simulink model "MOdel"  (R2019a)
settings: Solver=VariableStepAuto  StartTime=0.0  StopTime=30  RelTol=1e-3
libraries: simulink x2, vrlib x2, mpcadaslib x1
settings Model: Creator=pawar  LastModifiedBy=pawar

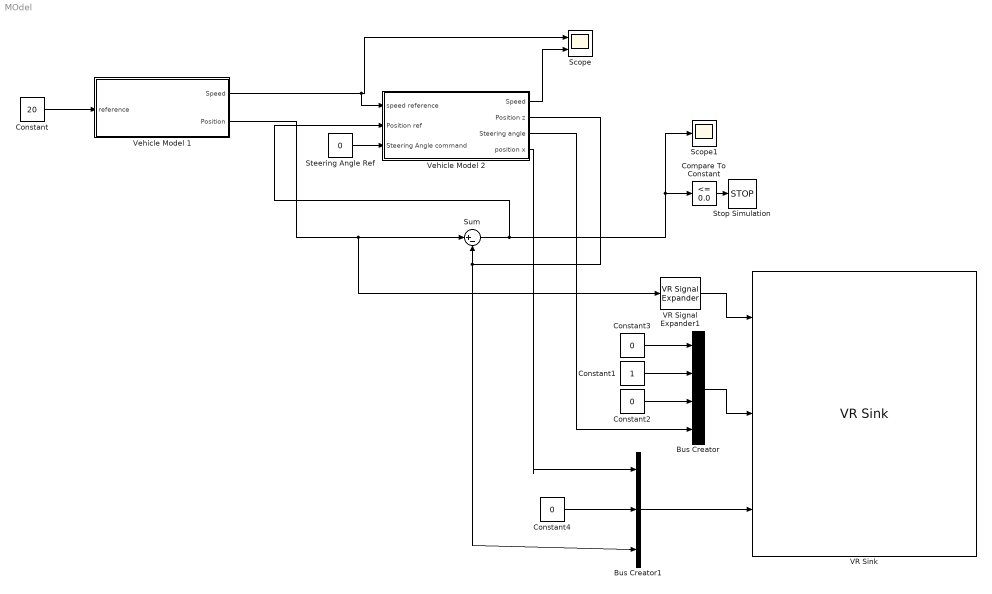
== system MOdel ==
  Bus Creator : BusCreator  Inputs=4
  Bus Creator1 : BusCreator  Inputs=3
  Compare To Constant : simulink/Logic and Bit Operations/Compare To Constant  relop=<=  const=0.0  OutDataTypeStr=boolean
  Constant : Constant  Value=20
  Constant1 : Constant
  Constant2 : Constant  Value=0
  Constant3 : Constant  Value=0
  Constant4 : Constant  Value=0
  Scope : Scope  NumInputPorts=2
  Scope1 : Scope
  Steering Angle Ref : Constant  Value=0
  Stop Simulation : Stop
  Sum : Sum  Inputs=|+-
  VR Signal Expander1 : vrlib/VR Signal Expander  outwidth=3  outidx=[3]
      settings: SourceProductName=Simulink
  VR Sink : vrlib/VR Sink  InstantiateOnLoad=on  SampleTime=0.1  ViewEnable=on  RemoteChange=off  RemoteView=off  FieldsWritten=Car_Red.translation.3.1.1.double#Car_Blue.rotation.4.1.1.double#Car_Blue.translation.3.1.1.double  WorldFileName=PlatoonWorld.WRL  AutoView=off  VideoDimensions=[]  AllowVariableSize=off
      settings: SourceProductName=Simulink
  Vehicle Model 1 : Subsystem  mask{Parameter3=[], Value=10, Value_1=20}
      mask prompts: Value "Initial Speed"; Value_1 "Initail Position"
      mask TypeOptions Value:
      | Initial Speed
      | /Value
      mask TypeOptions Value_1: Initial Position/Value
  Vehicle Model 2 : Subsystem  mask{Parameter3=[], Value=5, V=0}
      mask prompts: Value "Initial Speed"; V "Initial Position"
      mask TypeOptions Value:
      | Initial Speed
      | /Value
      mask TypeOptions V: Initial Position z/Value
  wires:
  Constant/1 -> Vehicle Model 1/1(reference)
  Vehicle Model 1/1(Speed) -> Vehicle Model 2/1(speed reference), Scope/1
  Vehicle Model 1/2("Position ") -> VR Signal Expander1/1, Sum/1
  Vehicle Model 2/1(Speed) -> Scope/2
  Vehicle Model 2/2("Position z ") -> Bus Creator1/3, Sum/2
  Sum/1 -> Vehicle Model 2/2("Position ref "), Compare To Constant/1, Scope1/1
  Compare To Constant/1 -> Stop Simulation/1
  Steering Angle Ref/1 -> Vehicle Model 2/3(Steering Angle command)
  VR Signal Expander1/1 -> VR Sink/1
  Bus Creator1/1 -> VR Sink/3
  Vehicle Model 2/3(Steering angle) -> Bus Creator/4
  Bus Creator/1 -> VR Sink/2
  Constant1/1 -> Bus Creator/2
  Constant3/1 -> Bus Creator/1
  Constant2/1 -> Bus Creator/3
  Constant4/1 -> Bus Creator1/2
  Vehicle Model 2/4(position x) -> Bus Creator1/1

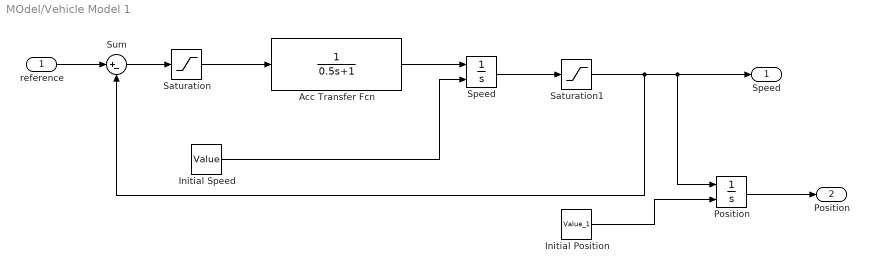
== system MOdel/Vehicle Model 1 ==
  reference : Inport
  Acc Transfer Fcn : TransferFcn  Denominator=[0.5 1]
  Initial Position : Constant  Value=Value_1
  "Initial Speed " : Constant  Value=Value
  Position : Integrator  InitialConditionSource=external
  Saturation : Saturate  UpperLimit=2  LowerLimit=-3
  Saturation1 : Saturate  UpperLimit=inf  LowerLimit=0
  "Speed " : Integrator  InitialConditionSource=external
  Sum : Sum  Inputs=|+-
  Speed : Outport
  "Position " : Outport  Port=2
  wires:
  Saturation1/1 -> Sum/2, Speed/1, Position/1
  Saturation/1 -> Acc Transfer Fcn/1
  "Initial Speed "/1 -> "Speed "/2
  Position/1 -> "Position "/1
  Sum/1 -> Saturation/1
  reference/1 -> Sum/1
  Acc Transfer Fcn/1 -> "Speed "/1
  Initial Position/1 -> Position/2
  "Speed "/1 -> Saturation1/1

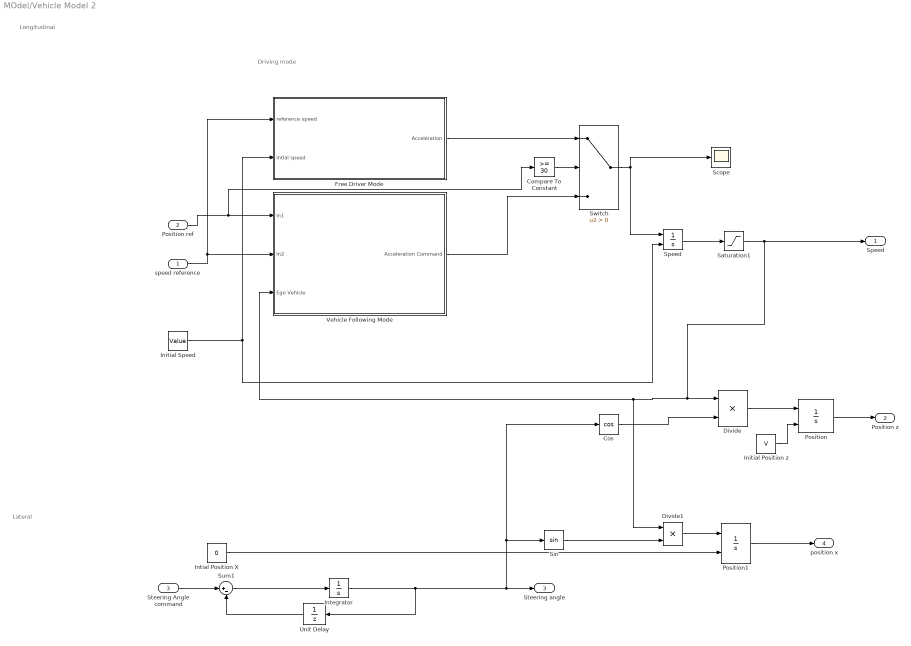
== system MOdel/Vehicle Model 2 ==
  note: Driving mode
  note: Lateral
  note: Longitudinal
  speed reference : Inport
  "Position ref " : Inport  Port=2
  Steering Angle command : Inport  Port=3
  Compare To Constant : simulink/Logic and Bit Operations/Compare To Constant  relop=>=  const=30  OutDataTypeStr=boolean
  Cos : Trigonometry  Operator=cos
  Divide : Product  Inputs=**
  Divide1 : Product  Inputs=**
  Free Driver Mode : Subsystem
  Initial Position z : Constant  Value=V
  "Initial Speed " : Constant  Value=Value
  Integrator : Integrator
  "Intial Position X " : Constant  Value=0
  Position : Integrator  InitialConditionSource=external
  Position1 : Integrator  InitialConditionSource=external
  Saturation1 : Saturate  UpperLimit=inf  LowerLimit=0
  Scope : Scope
  Sin : Trigonometry
  "Speed " : Integrator  InitialConditionSource=external
  Sum1 : Sum  Inputs=|+-
  Switch : Switch  Criteria=u2 > Threshold
  Unit Delay : UnitDelay  SampleTime=-1  HasFrameUpgradeWarning=on
  Vehicle Following Mode : Subsystem
  Speed : Outport
  "Position z " : Outport  Port=2
  Steering angle : Outport  Port=3
  position x : Outport  Port=4
  wires:
  "Initial Speed "/1 -> Free Driver Mode/2(Intial speed), "Speed "/2
  Position/1 -> "Position z "/1
  Initial Position z/1 -> Position/2
  "Speed "/1 -> Saturation1/1
  Saturation1/1 -> Vehicle Following Mode/3(Ego Vehicle), Divide1/1, Divide/1, Speed/1
  Integrator/1 -> Unit Delay/1, Cos/1, Sin/1, Steering angle/1
  Steering Angle command/1 -> Sum1/1
  Sum1/1 -> Integrator/1
  Unit Delay/1 -> Sum1/2
  Position1/1 -> position x/1
  "Intial Position X "/1 -> Position1/2
  Cos/1 -> Divide/2
  Divide/1 -> Position/1
  Sin/1 -> Divide1/2
  Divide1/1 -> Position1/1
  "Position ref "/1 -> Compare To Constant/1, Vehicle Following Mode/1(In1)
  speed reference/1 -> Free Driver Mode/1(reference speed), Vehicle Following Mode/2(In2)
  Switch/1 -> "Speed "/1, Scope/1
  Vehicle Following Mode/1(Acceleration Command) -> Switch/3
  Free Driver Mode/1(Acceleration) -> Switch/1
  Compare To Constant/1 -> Switch/2

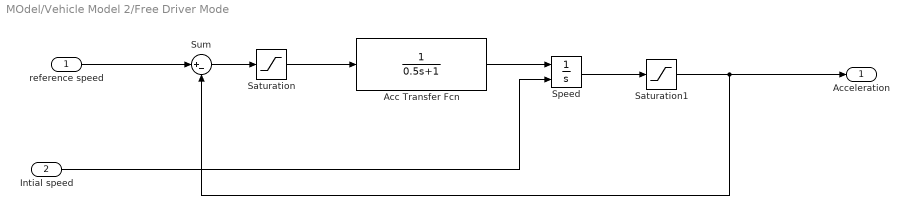
== system MOdel/Vehicle Model 2/Free Driver Mode ==
  reference speed : Inport
  Intial speed : Inport  Port=2
  Acc Transfer Fcn : TransferFcn  Denominator=[0.5 1]
  Saturation : Saturate  UpperLimit=2  LowerLimit=-3
  Saturation1 : Saturate  UpperLimit=inf  LowerLimit=0
  "Speed " : Integrator  InitialConditionSource=external
  Sum : Sum  Inputs=|+-
  Acceleration : Outport
  wires:
  "Speed "/1 -> Saturation1/1
  Acc Transfer Fcn/1 -> "Speed "/1
  reference speed/1 -> Sum/1
  Saturation/1 -> Acc Transfer Fcn/1
  Saturation1/1 -> Acceleration/1, Sum/2
  Sum/1 -> Saturation/1
  Intial speed/1 -> "Speed "/2

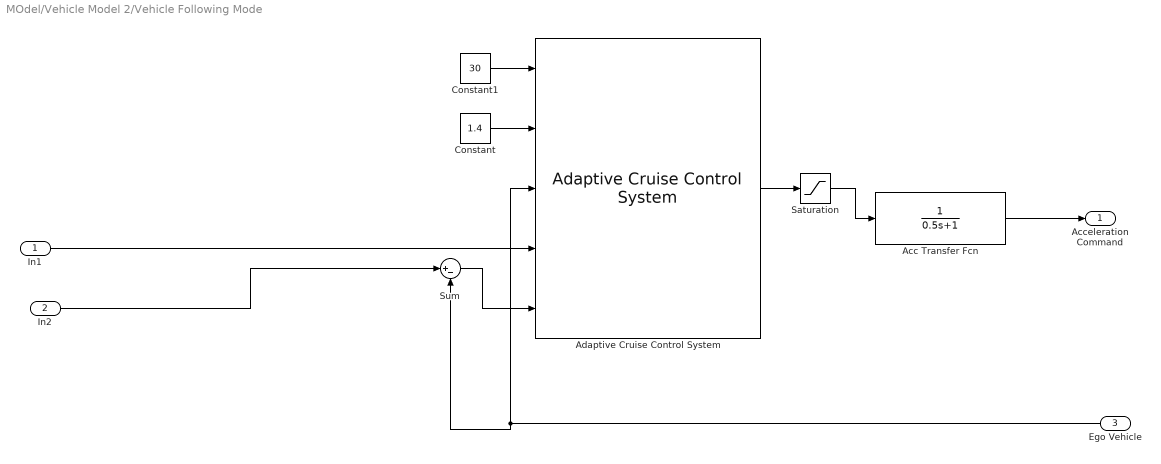
== system MOdel/Vehicle Model 2/Vehicle Following Mode ==
  In1 : Inport
  In2 : Inport  Port=2
  Ego Vehicle : Inport  Port=3
  Acc Transfer Fcn : TransferFcn  Denominator=[0.5 1]
  Adaptive Cruise Control System : mpcadaslib/Adaptive Cruise Control System  EgoModel=tf(1,[0.5,1,0])  InitialEgoVelocity=30  DefaultSpacing=5  MaxVelocity=50  MinAcceleration=-3  amin_ext=off  MaxAcceleration=2  amax_ext=off  Ts=0.5  PredictionHorizon=200  ControllerBehavior=0.580  suboptimal=off  maxiter=10  datatypeopt=double  optmode=off  trackmode=off
      settings: SourceProductName=MATLAB Runtime - Model Predictive Control Toolbox Addin  SourceProductBaseCode=Missing
  Constant : Constant  Value=1.4
  Constant1 : Constant  Value=30
  Saturation : Saturate  UpperLimit=2  LowerLimit=-3
  Sum : Sum  Inputs=|+-
  Acceleration Command : Outport
  wires:
  Saturation/1 -> Acc Transfer Fcn/1
  In2/1 -> Sum/1
  Adaptive Cruise Control System/1 -> Saturation/1
  Constant1/1 -> Adaptive Cruise Control System/1
  Ego Vehicle/1 -> Sum/2, Adaptive Cruise Control System/3
  Sum/1 -> Adaptive Cruise Control System/5
  Acc Transfer Fcn/1 -> Acceleration Command/1
  Constant/1 -> Adaptive Cruise Control System/2
  In1/1 -> Adaptive Cruise Control System/4
